simulink model "new_version_with_correct_eq"  (R2022a)
settings: Solver=VariableStepAuto  StartTime=0.0  StopTime=15  RelTol=1e-6
undefined symbols (not defined in the file or in its folder): A, A2, B, B2, C, C2, D, D2, g, l, m, M, Q1, Q2
libraries: cstblocks x3
settings Model: Creator=Lukáš Kozel  LastModifiedBy=uzivatel
settings SolverCC: AlgebraicLoopSolver=LineSearch
settings DebuggingCC: UnconnectedInputMsg=warning  UnconnectedOutputMsg=warning  UnconnectedLineMsg=warning  SFMachineParentedDataDiag=warning

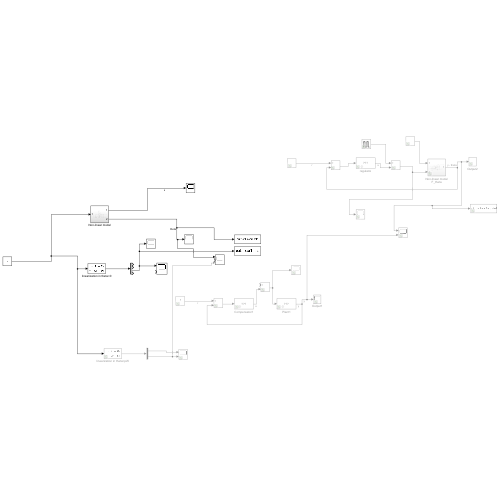
[thumbnail: Simulink's stored preview of the top-level diagram]
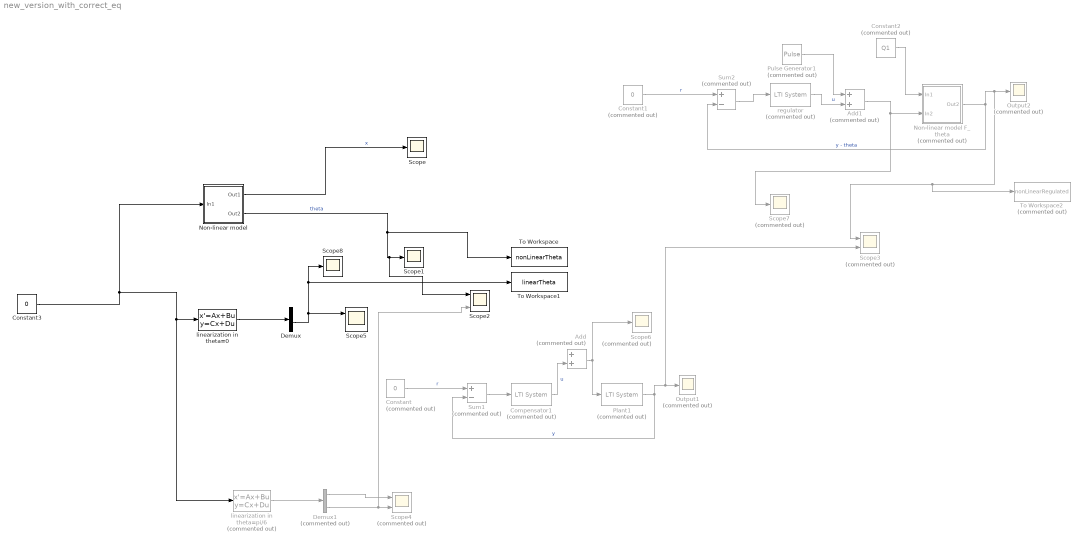
== system new_version_with_correct_eq ==
  Add : Sum  Commented=on
  Add1 : Sum  Commented=on
  Compensator1 : cstblocks/LTI System  Commented=on  sys=regulator  IC=[]
  Constant : Constant  Commented=on  Value=0
  Constant1 : Constant  Commented=on  Value=0
  Constant2 : Constant  Commented=on  Value=Q1
  Constant3 : Constant  Value=0
  Demux : Demux
  Demux1 : Demux  Commented=on  Outputs=2
  "Non-linear model " : Subsystem
  Non-linear model F_theta : Subsystem  Commented=on
  Output1 : Scope  Commented=on
  Output2 : Scope  Commented=on
  Plant1 : cstblocks/LTI System  Commented=on  sys=F_theta  IC=[]
  Pulse Generator1 : DiscretePulseGenerator  Commented=on  PulseType=Time based  Amplitude=Q2  Period=10  PulseWidth=0.001  PhaseDelay=5
  Scope : Scope
  Scope1 : Scope
  Scope2 : Scope  NumInputPorts=3
  Scope3 : Scope  Commented=on  NumInputPorts=2
  Scope4 : Scope  Commented=on  NumInputPorts=2
  Scope5 : Scope  NumInputPorts=2
  Scope6 : Scope  Commented=on
  Scope7 : Scope  Commented=on
  Scope8 : Scope
  Sum1 : Sum  Commented=on  Inputs=+-  InputSameDT=on  SaturateOnIntegerOverflow=on  OutDataTypeStr=Inherit: Same as first input
  Sum2 : Sum  Commented=on  Inputs=+-  InputSameDT=on  SaturateOnIntegerOverflow=on  OutDataTypeStr=Inherit: Same as first input
  To Workspace : ToWorkspace  VariableName=nonLinearTheta  SaveFormat=Timeseries  SampleTime=-1
  To Workspace1 : ToWorkspace  VariableName=linearTheta  SaveFormat=Timeseries  SampleTime=-1
  To Workspace2 : ToWorkspace  Commented=on  VariableName=nonLinearRegulated  SaveFormat=Timeseries  SampleTime=-1
  linearization in theta=0 : StateSpace  A=A  B=B  C=C  D=D  InitialCondition=[0,0,pi/16,0]
  linearization in theta=pi/6 : StateSpace  Commented=on  A=A2  B=B2  C=C2  D=D2  InitialCondition=0
  regulator : cstblocks/LTI System  Commented=on  sys=regulator  IC=[]
  wires:
  Constant3/1 -> linearization in theta=pi/6/1, linearization in theta=0/1, "Non-linear model "/1(In1)
  linearization in theta=0/1 -> Demux/1
  "Non-linear model "/1(Out1) -> Scope/1  "x"
  "Non-linear model "/2(Out2) -> Scope2/1, Scope1/1, To Workspace/1  "theta"
  Constant/1 -> Sum1/1  "r"
  Plant1/1 -> Scope3/2, Output1/1, Sum1/2  "y"
  Sum1/1 -> Compensator1/1
  Compensator1/1 -> Add/2  "u"
  Add/1 -> Plant1/1, Scope6/1
  Non-linear model F_theta/1(Out2) -> To Workspace2/1, Scope3/1, Output2/1, Sum2/2  "y - theta"
  Constant1/1 -> Sum2/1  "r"
  Sum2/1 -> regulator/1
  Add1/1 -> Scope7/1, Non-linear model F_theta/2(In2)
  regulator/1 -> Add1/2  "u"
  Pulse Generator1/1 -> Add1/1
  Constant2/1 -> Non-linear model F_theta/1(In1)
  Demux1/1 -> Scope4/1
  linearization in theta=pi/6/1 -> Demux1/1
  Demux1/2 -> Scope2/3, Scope4/2
  Demux/3 -> To Workspace1/1, Scope8/1, Scope5/1

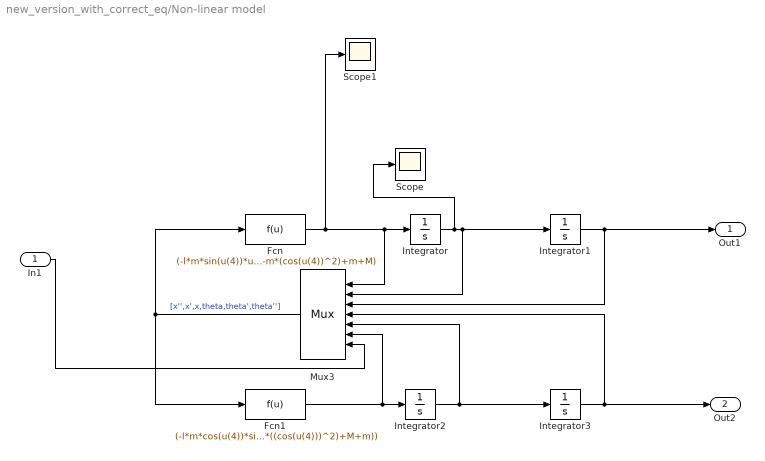
== system new_version_with_correct_eq/Non-linear model  ==
  In1 : Inport
  Fcn : Fcn  Expr=(-l*m*sin(u(4))*u(5)^2+u(7)-m*g*cos(u(4))*sin(u(4)))/(-m*(cos(u(4))^2)+m+M)
  Fcn1 : Fcn  Expr=(-l*m*cos(u(4))*sin(u(4))*u(5)^2+u(7)*cos(u(4))-g*m*sin(u(4))-M*g*sin(u(4)))/(l*(-m*((cos(u(4)))^2)+M+m))
  Integrator : Integrator
  Integrator1 : Integrator
  Integrator2 : Integrator
  Integrator3 : Integrator  InitialCondition=pi/16
  Mux3 : Mux  Inputs=7
      settings: DisplayOption=signals
  Scope : Scope
  Scope1 : Scope
  Out1 : Outport
  Out2 : Outport  Port=2
  wires:
  Integrator/1 -> Scope/1, Mux3/2, Integrator1/1
  Fcn1/1 -> Mux3/6, Integrator2/1
  Mux3/1 -> Fcn/1, Fcn1/1  "[x'',x',x,theta,theta',theta'']"
  Integrator1/1 -> Out1/1, Mux3/3
  Integrator3/1 -> Out2/1, Mux3/4
  Integrator2/1 -> Mux3/5, Integrator3/1
  Fcn/1 -> Mux3/1, Integrator/1, Scope1/1
  In1/1 -> Mux3/7

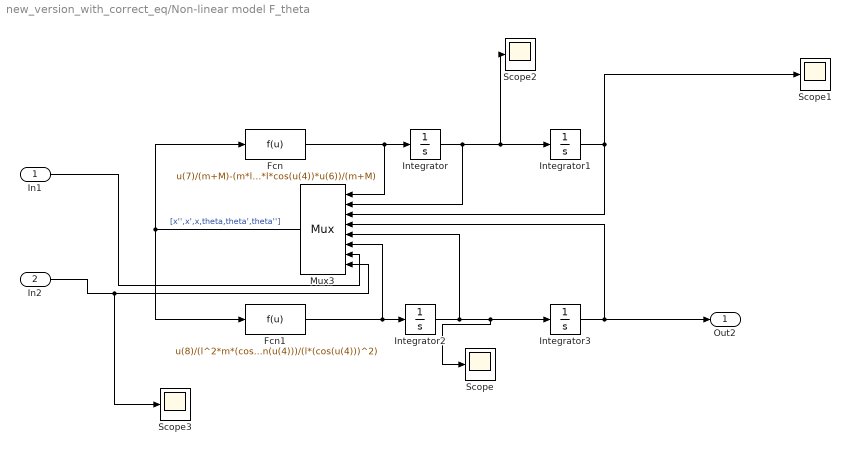
== system new_version_with_correct_eq/Non-linear model F_theta ==
  In1 : Inport
  In2 : Inport  Port=2
  Fcn : Fcn  Expr=u(7)/(m+M)-(m*l*sin(u(4))*(u(5))^2)/(m+M)+(m*l*cos(u(4))*u(6))/(m+M)
  Fcn1 : Fcn  Expr=u(8)/(l^2*m*(cos(u(4)))^2)+(u(1))/(l*cos(u(4)))+(sin(u(4))*(u(4))^2)/(cos(u(4)))-(g*sin(u(4)))/(l*(cos(u(4)))^2)
  Integrator : Integrator
  Integrator1 : Integrator
  Integrator2 : Integrator
  Integrator3 : Integrator  InitialCondition=pi/6
  Mux3 : Mux  Inputs=8
      settings: DisplayOption=signals
  Scope{,1..3} (4 alike) : Scope
  Out2 : Outport
  wires:
  Integrator/1 -> Mux3/2, Scope2/1, Integrator1/1
  Fcn1/1 -> Mux3/6, Integrator2/1
  In2/1 -> Scope3/1, Mux3/8
  Mux3/1 -> Fcn/1, Fcn1/1  "[x'',x',x,theta,theta',theta'']"
  Integrator1/1 -> Scope1/1, Mux3/3
  Integrator3/1 -> Out2/1, Mux3/4
  Integrator2/1 -> Mux3/5, Scope/1, Integrator3/1
  Fcn/1 -> Mux3/1, Integrator/1
  In1/1 -> Mux3/7
